simulink model "teste_odometria_udp_lidarloc"  (R2024a)
settings: configuration reference "SharedConfig" (kept outside this file)
model workspace (MAT data in the model file):
  mdlWSDbList = "tramontina_database_curtis.dbc"
undefined symbols (not defined in the file): Down, Pull
libraries: tramontina_database_curtislib x6, speedgoatlib_IO60X_IO69X x1, speedgoatlib_IO691 x1, slrealtimeiplib x1, slrealtimeptplib x1
settings Model: DataDictionary=configuration_dictionary.sldd  Creator=matlab.cut  LastModifiedBy=matlab.cut
settings ConfigSetRef: SourceName=SharedConfig

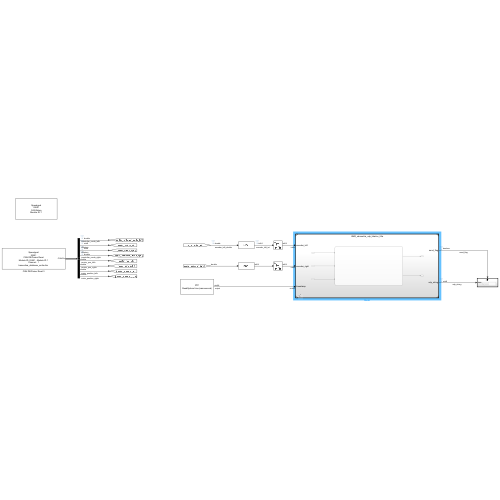
[thumbnail: Simulink's stored preview of the top-level diagram]
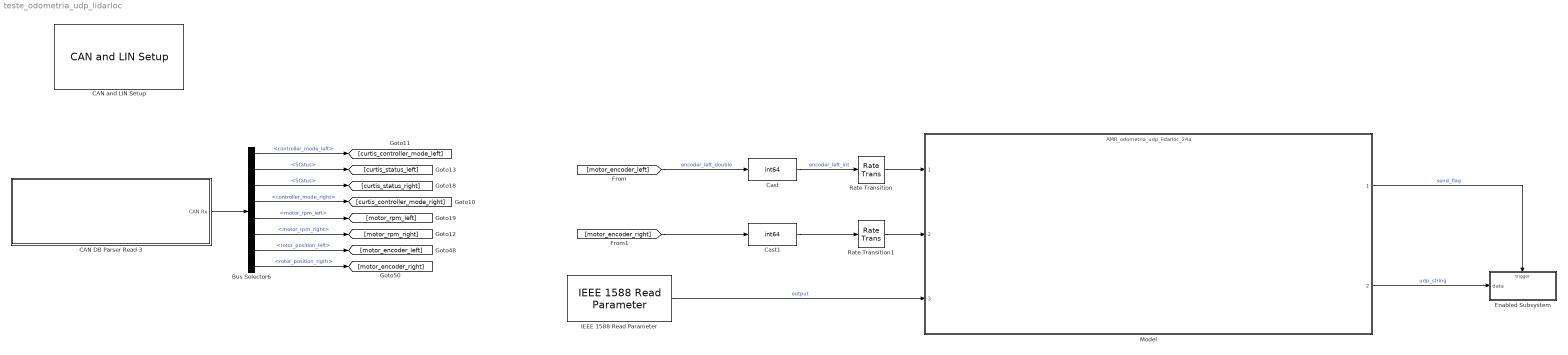
== system teste_odometria_udp_lidarloc ==
  Bus Selector6 : BusSelector  OutputSignals=ID1830_controller_status_left.controller_mode_left,ID1830_controller_status_left.MessageStatus.Status,ID1831_controller_status_right.MessageStatus.Status,ID1831_controller_status_right.controller_mode_right,ID422_curtis_feedback_message_left.motor_rpm_left,ID423_curtis_feedback_message_right.motor_rpm_right,ID934_curtis_encoder_left.rotor_position_left,ID935_curtis_encoder_right.rotor_position_rigth
  CAN DB Parser Read 3 : Subsystem
      settings: OpenFcn=sg_can.OpenFcnRead;
      mask Help: eval('sg.utils.help.show(''io_main/refentry_ref_can_ofa_parsing_read'');')
      mask Display: disp('Speedgoat\nIO691\nCAN DB Parser Read\nModule ID: IO691 - Module ID 1\nChannel:  1\ntramontina_database_curtis.dbc ');
  "CAN and LIN Setup " : speedgoatlib_IO691/CAN and LIN Setup   moduleInitValues="[691    1    1   -1   -1]"  id=1  moduleType=IO691  pciSlot=-1  canChn1=CAN (HS)  canChn2=Disabled  canChn3=Disabled  canChn4=Disabled  linChn1=Disabled  linChn2=Disabled  canInitStructArray=[]  canTermStructArray=[]  gpioChnx=Disabled  canChn1InitValues="[2   2   8   1  16   3  19   2   2   5   2   0]"  arbBdrChn1=500 kBaud  clockDividerChn1=Enable  arbManBdrChn1=[8,1,16,3]  fdBdrChn1=5.0 MBaud  fdManBdrChn1=[2,2,5,2]  termResistor1=off  canChn2InitValues="[1   0   2   8  31   8  19   2   2   5   2   0]"  arbBdrChn2=1.0 MBaud  clockDividerChn2=Enable  arbManBdrChn2=[2,8,31,8]  fdBdrChn2=5.0 MBaud  fdManBdrChn2=[2,2,5,2]  termResistor2=off  canChn3InitValues="[1   0   2   8  31   8  19   2   2   5   2   0]"  arbBdrChn3=1.0 MBaud  clockDividerChn3=Enable  arbManBdrChn3=[2,8,31,8]  fdBdrChn3=5.0 MBaud  fdManBdrChn3=[2,2,5,2]  termResistor3=off  canChn4InitValues="[1   0   2   8  31   8  19   2   2   5   2   0]"  arbBdrChn4=1.0 MBaud  clockDividerChn4=Enable  arbManBdrChn4=[2,8,31,8]  fdBdrChn4=5.0 MBaud  fdManBdrChn4=[2,2,5,2]  termResistor4=off  linChn1InitValues="[0  9600]"  linBtrChn1=9600  linChn2InitValues="[0  9600]"  linBtrChn2=9600  doInitTermStruct="[0  5  0  0  0]"  parDoChannels=[1 2]  parDoVoltage=5  parDoInitValues=0  parDoReset=1  parNumOfDoS=0  parDiChannels=[3 4]  parDiVoltage=5  parDiPull=Pull-Down
      settings: LibrarySourceBlock=speedgoatlib_IO602_IO691/CAN and LIN Setup
  Cast : DataTypeConversion  OutDataTypeStr=int64  SaturateOnIntegerOverflow=off  RndMeth=Floor
  Cast1 : DataTypeConversion  OutDataTypeStr=int64  SaturateOnIntegerOverflow=off  RndMeth=Floor
  Enabled Subsystem : Subsystem  TreatAsAtomicUnit=on
  IEEE 1588 Read Parameter : slrealtimeptplib/IEEE 1588 Read Parameter  Priority=1  ID=1  param=1. System time (nanosecond)  sample_time=-1
  Model : ModelReference  ModelNameDialog=AMR_odometria_udp_lidarloc_24a.slx  SimulationMode=Normal  ModelReferenceVersion=1.9
  Rate Transition : RateTransition
  Rate Transition1 : RateTransition
  wires:
  Bus Selector6/3 -> [curtis_status_right]  "<Status>"
  Bus Selector6/1 -> [curtis_controller_mode_left]  "<controller_mode_left>"
  Bus Selector6/5 -> [motor_rpm_left]  "<motor_rpm_left>"
  Bus Selector6/2 -> [curtis_status_left]  "<Status>"
  CAN DB Parser Read 3/1(CAN Rx) -> Bus Selector6/1
  Bus Selector6/8 -> [motor_encoder_right]  "<rotor_position_rigth>"
  Bus Selector6/6 -> [motor_rpm_right]  "<motor_rpm_right>"
  Bus Selector6/7 -> [motor_encoder_left]  "<rotor_position_left>"
  Bus Selector6/4 -> [curtis_controller_mode_right]  "<controller_mode_right>"
  [motor_encoder_left] -> Cast/1  "encoder_left_double"
  [motor_encoder_right] -> Cast1/1
  Model/1 -> Enabled Subsystem/Trigger  "send_flag"
  Model/2 -> Enabled Subsystem/1(data)  "udp_string"
  IEEE 1588 Read Parameter/1 -> Model/3  "output"
  Cast/1 -> Rate Transition/1  "encoder_left_int"
  Cast1/1 -> Rate Transition1/1
  Rate Transition/1 -> Model/1
  Rate Transition1/1 -> Model/2

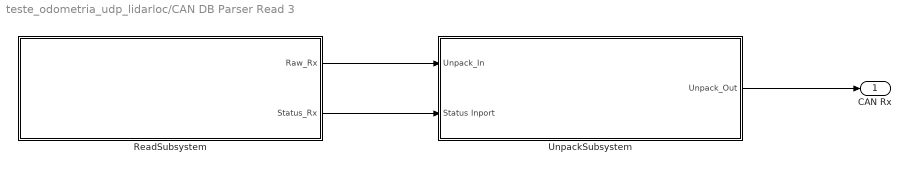
== system teste_odometria_udp_lidarloc/CAN DB Parser Read 3 ==
  ReadSubsystem : Subsystem
  UnpackSubsystem : Subsystem
  CAN Rx : Outport
  wires:
  ReadSubsystem/1(Raw_Rx) -> UnpackSubsystem/1(Unpack_In)
  ReadSubsystem/2(Status_Rx) -> UnpackSubsystem/2(Status Inport)
  UnpackSubsystem/1(Unpack_Out) -> CAN Rx/1

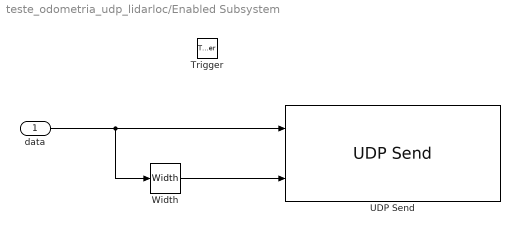
== system teste_odometria_udp_lidarloc/Enabled Subsystem ==
  data : Inport
  Trigger : TriggerPort  VariantControl=(inherit)  PortDimensions=1
  UDP Send : slrealtimeiplib/UDP Send  useHostTargetConn=off  toAddress='10.200.83.69'  toPort=34  sampleTime=-1  enableMessage=off
  Width : Width
  wires:
  data/1 -> UDP Send/1, Width/1
  Width/1 -> UDP Send/2

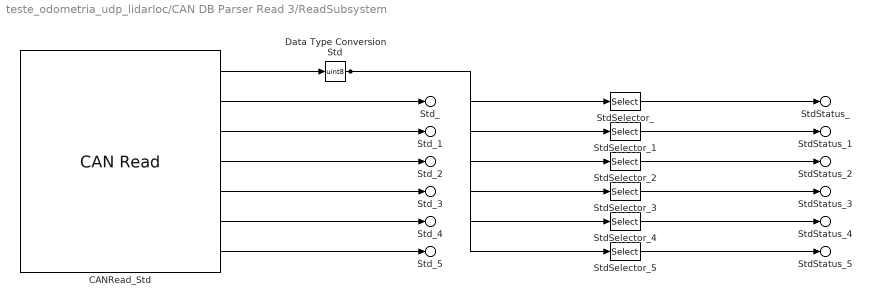
== system teste_odometria_udp_lidarloc/CAN DB Parser Read 3/ReadSubsystem ==
  CANRead_Std : speedgoatlib_IO60X_IO69X/CAN/CAN Read   moduleType=IO691  id=1  channel=1  canType=CAN (HS)  messageType=CAN (HS)  useBusOut=on  HasMulRead=Specify by IDs  MsgIDlist="[422   423   934   935  1830  1831]"  isEFF=off  LabelInHex=off  enableInput=off  initValues=[691 1 0.03 0 1 1 0 1 2 0 6 422 423 934 935 1830 1831]  ts=30e-3
  Data Type ConversionStd : DataTypeConversion  OutDataTypeStr=uint8  SaturateOnIntegerOverflow=off  RndMeth=Floor
  StdSelector_ : Selector  IndexOptions=Index vector (dialog)  Indices=1  OutputSizes=1
  StdSelector_1 : Selector  IndexOptions=Index vector (dialog)  Indices=2  OutputSizes=1
  StdSelector_2 : Selector  IndexOptions=Index vector (dialog)  Indices=3  OutputSizes=1
  StdSelector_3 : Selector  IndexOptions=Index vector (dialog)  Indices=4  OutputSizes=1
  StdSelector_4 : Selector  IndexOptions=Index vector (dialog)  Indices=5  OutputSizes=1
  StdSelector_5 : Selector  IndexOptions=Index vector (dialog)  Indices=6  OutputSizes=1
  Std_ : Outport  PortName=Raw_Rx  Element=Std.ID422
  Std_1 : Outport  PortName=Raw_Rx  Element=Std.ID423
  Std_2 : Outport  PortName=Raw_Rx  Element=Std.ID934
  Std_3 : Outport  PortName=Raw_Rx  Element=Std.ID935
  Std_4 : Outport  PortName=Raw_Rx  Element=Std.ID1830
  Std_5 : Outport  PortName=Raw_Rx  Element=Std.ID1831
  StdStatus_ : Outport  Port=2  PortName=Status_Rx  Element=Std.ID422
  StdStatus_1 : Outport  Port=2  PortName=Status_Rx  Element=Std.ID423
  StdStatus_2 : Outport  Port=2  PortName=Status_Rx  Element=Std.ID934
  StdStatus_3 : Outport  Port=2  PortName=Status_Rx  Element=Std.ID935
  StdStatus_4 : Outport  Port=2  PortName=Status_Rx  Element=Std.ID1830
  StdStatus_5 : Outport  Port=2  PortName=Status_Rx  Element=Std.ID1831
  wires:
  CANRead_Std/1 -> Data Type ConversionStd/1
  CANRead_Std/2 -> Std_/1
  CANRead_Std/3 -> Std_1/1
  CANRead_Std/4 -> Std_2/1
  CANRead_Std/5 -> Std_3/1
  CANRead_Std/6 -> Std_4/1
  CANRead_Std/7 -> Std_5/1
  Data Type ConversionStd/1 -> StdSelector_/1, StdSelector_1/1, StdSelector_2/1, StdSelector_3/1, StdSelector_4/1, StdSelector_5/1
  StdSelector_/1 -> StdStatus_/1
  StdSelector_1/1 -> StdStatus_1/1
  StdSelector_2/1 -> StdStatus_2/1
  StdSelector_3/1 -> StdStatus_3/1
  StdSelector_4/1 -> StdStatus_4/1
  StdSelector_5/1 -> StdStatus_5/1

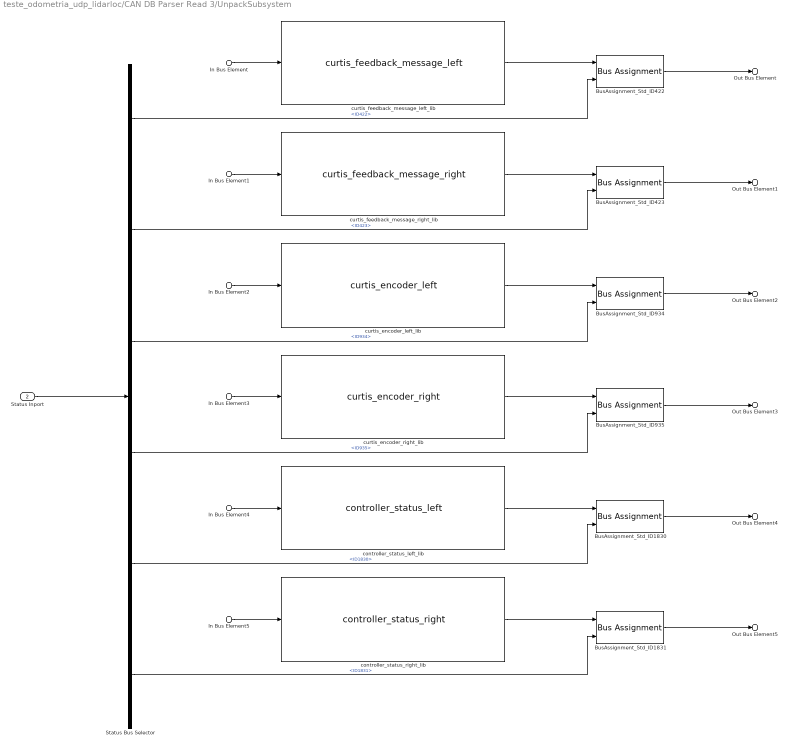
== system teste_odometria_udp_lidarloc/CAN DB Parser Read 3/UnpackSubsystem ==
  In Bus Element : Inport  PortName=Unpack_In  Element=Std.ID422
  In Bus Element1 : Inport  PortName=Unpack_In  Element=Std.ID423
  In Bus Element2 : Inport  PortName=Unpack_In  Element=Std.ID934
  In Bus Element3 : Inport  PortName=Unpack_In  Element=Std.ID935
  In Bus Element4 : Inport  PortName=Unpack_In  Element=Std.ID1830
  In Bus Element5 : Inport  PortName=Unpack_In  Element=Std.ID1831
  Status Inport : Inport  Port=2
  BusAssignment_Std_ID{422..423,934..935,1830..1831} (6 alike) : BusAssignment  AssignedSignals=MessageStatus.Status
  Status Bus Selector : BusSelector  OutputSignals=Std.ID422,Std.ID423,Std.ID934,Std.ID935,Std.ID1830,Std.ID1831
  controller_status_left_lib : tramontina_database_curtislib/CAN unpack/controller_status_left  SystemSampleTime=-1  VariantActivationTime=update diagram  AllowFlexibleInterface=on  Latency=0  AutoFrameSizeCalculation=off
  controller_status_right_lib : tramontina_database_curtislib/CAN unpack/controller_status_right  SystemSampleTime=-1  VariantActivationTime=update diagram  AllowFlexibleInterface=on  Latency=0  AutoFrameSizeCalculation=off
  curtis_encoder_left_lib : tramontina_database_curtislib/CAN unpack/curtis_encoder_left  SystemSampleTime=-1  VariantActivationTime=update diagram  AllowFlexibleInterface=on  Latency=0  AutoFrameSizeCalculation=off
  curtis_encoder_right_lib : tramontina_database_curtislib/CAN unpack/curtis_encoder_right  SystemSampleTime=-1  VariantActivationTime=update diagram  AllowFlexibleInterface=on  Latency=0  AutoFrameSizeCalculation=off
  curtis_feedback_message_left_lib : tramontina_database_curtislib/CAN unpack/curtis_feedback_message_left  SystemSampleTime=-1  VariantActivationTime=update diagram  AllowFlexibleInterface=on  Latency=0  AutoFrameSizeCalculation=off
  curtis_feedback_message_right_lib : tramontina_database_curtislib/CAN unpack/curtis_feedback_message_right  SystemSampleTime=-1  VariantActivationTime=update diagram  AllowFlexibleInterface=on  Latency=0  AutoFrameSizeCalculation=off
  Out Bus Element : Outport  PortName=Unpack_Out  Element=ID422_curtis_feedback_message_left
  Out Bus Element1 : Outport  PortName=Unpack_Out  Element=ID423_curtis_feedback_message_right
  Out Bus Element2 : Outport  PortName=Unpack_Out  Element=ID934_curtis_encoder_left
  Out Bus Element3 : Outport  PortName=Unpack_Out  Element=ID935_curtis_encoder_right
  Out Bus Element4 : Outport  PortName=Unpack_Out  Element=ID1830_controller_status_left
  Out Bus Element5 : Outport  PortName=Unpack_Out  Element=ID1831_controller_status_right
  wires:
  In Bus Element/1 -> curtis_feedback_message_left_lib/1
  curtis_feedback_message_left_lib/1 -> BusAssignment_Std_ID422/1
  BusAssignment_Std_ID422/1 -> Out Bus Element/1
  In Bus Element1/1 -> curtis_feedback_message_right_lib/1
  curtis_feedback_message_right_lib/1 -> BusAssignment_Std_ID423/1
  BusAssignment_Std_ID423/1 -> Out Bus Element1/1
  In Bus Element2/1 -> curtis_encoder_left_lib/1
  curtis_encoder_left_lib/1 -> BusAssignment_Std_ID934/1
  BusAssignment_Std_ID934/1 -> Out Bus Element2/1
  In Bus Element3/1 -> curtis_encoder_right_lib/1
  curtis_encoder_right_lib/1 -> BusAssignment_Std_ID935/1
  BusAssignment_Std_ID935/1 -> Out Bus Element3/1
  In Bus Element4/1 -> controller_status_left_lib/1
  controller_status_left_lib/1 -> BusAssignment_Std_ID1830/1
  BusAssignment_Std_ID1830/1 -> Out Bus Element4/1
  In Bus Element5/1 -> controller_status_right_lib/1
  controller_status_right_lib/1 -> BusAssignment_Std_ID1831/1
  BusAssignment_Std_ID1831/1 -> Out Bus Element5/1
  Status Inport/1 -> Status Bus Selector/1
  Status Bus Selector/1 -> BusAssignment_Std_ID422/2  "<ID422>"
  Status Bus Selector/2 -> BusAssignment_Std_ID423/2  "<ID423>"
  Status Bus Selector/3 -> BusAssignment_Std_ID934/2  "<ID934>"
  Status Bus Selector/4 -> BusAssignment_Std_ID935/2  "<ID935>"
  Status Bus Selector/5 -> BusAssignment_Std_ID1830/2  "<ID1830>"
  Status Bus Selector/6 -> BusAssignment_Std_ID1831/2  "<ID1831>"
